simulink model "Tank"  (R2013b)
settings: Solver=ode45  StartTime=0.0  StopTime=100.0  RelTol=1e-3
libraries: fuzblock x1
settings Model: Creator=Ahmed KH  LastModifiedBy=Ahmed KH
settings SolverCC: ZeroCrossControl=DisableAll

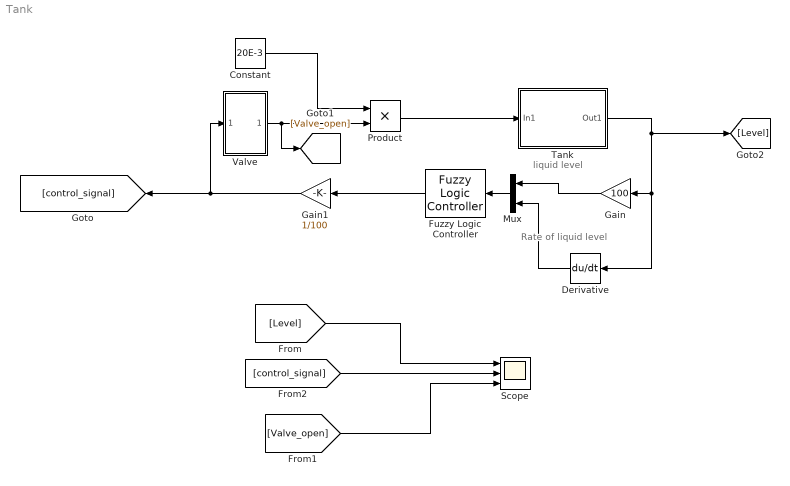
== system Tank ==
  note: Rate of
      | liquid level
  note: liquid level
  Constant : Constant  Value=20E-3
  Derivative : Derivative
  Fuzzy Logic Controller : fuzblock/Fuzzy Logic  Controller  fis=['Tank_level_system2.fis']
  Gain : Gain  Gain=100
  Gain1 : Gain  Gain=1/100
  Mux : Mux  Inputs=2
  Product : Product
  Scope : Scope  NumInputPorts=3
      settings: YMin=-5~-5~-5  YMax=5~5~5
  Tank : Subsystem
  Valve : Subsystem
  wires:
  Product/1 -> Tank/1(In1)
  Tank/1(Out1) -> [Level], Derivative/1, Gain/1
  Fuzzy Logic Controller/1 -> Gain1/1
  Valve/1(Out1) -> [Valve_open], Product/2
  Constant/1 -> Product/1
  Gain1/1 -> [control_signal], Valve/1(In1)
  Mux/1 -> Fuzzy Logic Controller/1
  Gain/1 -> Mux/1
  Derivative/1 -> Mux/2
  [Level] -> Scope/1
  [Valve_open] -> Scope/3
  [control_signal] -> Scope/2

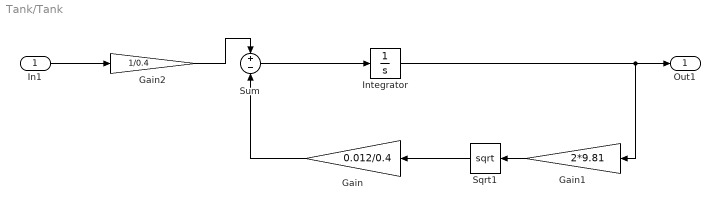
== system Tank/Tank ==
  In1 : Inport
  Gain : Gain  Gain=0.012/0.4
  Gain1 : Gain  Gain=2*9.81
  Gain2 : Gain  Gain=1/0.4
  Integrator : Integrator
  Sqrt1 : Sqrt  SaturateOnIntegerOverflow=on
  Sum : Sum  Inputs=+-
  Out1 : Outport
  wires:
  Integrator/1 -> Out1/1, Gain1/1
  Gain/1 -> Sum/2
  Sum/1 -> Integrator/1
  Sqrt1/1 -> Gain/1
  Gain1/1 -> Sqrt1/1
  Gain2/1 -> Sum/1
  In1/1 -> Gain2/1

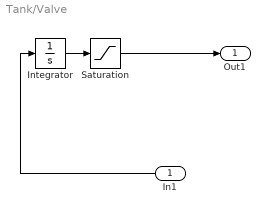
== system Tank/Valve ==
  In1 : Inport
  Integrator : Integrator
  Saturation : Saturate  UpperLimit=1  LowerLimit=0
  Out1 : Outport
  wires:
  Integrator/1 -> Saturation/1
  Saturation/1 -> Out1/1
  In1/1 -> Integrator/1
